simulink model "heli_q8"  (R2024b)
settings: Solver=ode1  StartTime=0.0  StopTime=5  FixedStep=0.002  RelTol=1e-3  EnableMultiTasking=on
PostLoadFcn:
  | qc_set_target_type(getConfigSet(bdroot, 'QUARC Default Target Configuration'));
values from neighbouring files (symbols this model uses):
  A_e = [0 1 0 0 0; 0 0 0 0 0; 0 0 0 1 0; 0 0 0 0 0; K_3 0 0 0 0]    [init_heli_3_10.m]
  Ad = sys_d.A    [init_heli_3_10.m]    (also in midlertidig.m)
  B_e = [0 0; 0 K_1; 0 0; K_2 0; 0 0]    [init_heli_3_10.m]
  Bd = sys_d.B    [init_heli_3_10.m]    (also in midlertidig.m)
  C_e = diag([1 1 1 1 1])    [init_heli_3_10.m]
  Cd = sys_d.C    [init_heli_3_10.m]    (also in midlertidig.m)
  Joystick_gain_x = 1    [init_heli_3_10.m]
  Joystick_gain_y = -1    [init_heli_3_10.m]
  L = place(A_e', C_e', p)'    [init_heli_3_10.m]
  Qd = diag([10^-5, 10^-3, 10^-5, 10^-3, 10^-5, 10^-3])    [init_heli_3_10.m]
  Rh = cov(Yh, 1)    [init_heli_3_10.m]    (also in midlertidig.m)
undefined symbols (not defined in the file or in its folder): HIL, qc_get_step_size
libraries: quarc_library x9
settings Model: SimulationMode=external  ExtModeTrigDuration=5000  Creator=Rchan  LastModifiedBy=Romeo
settings SolverCC: AlgebraicLoopSolver=TrustRegion  PositivePriorityOrder=on
settings DataIOCC: LimitDataPoints=on  SaveFormat=Array  SignalLoggingSaveFormat=ModelDataLogs  ReturnWorkspaceOutputs=off
settings OptimizationCC: ExpressionDepthLimit=2147483647  InitFltsAndDblsToZero=on  LifeSpan=inf
settings DebuggingCC: SaveWithParameterizedLinksMsg=none  UnderspecifiedInitializationDetection=Classic  MergeDetectMultiDrivingBlocksExec=none  SolverPrmCheckMsg=warning  MultiTaskDSMMsg=warning  MultiTaskCondExecSysMsg=none  FcnCallInpInsideContextMsg=warning  UnconnectedInputMsg=warning  UnconnectedOutputMsg=warning  UnconnectedLineMsg=warning  AllowSymbolicDim=off  StateNameClashWarn=warning  SFUnexpectedBacktrackingDiag=warning  SFNoUnconditionalDefaultTransitionDiag=warning  SFExecutionAtInitializationDiag=none  ArithmeticOperatorsInVariantConditions=warning
settings HardwareCC: ProdBitPerPointer=32  ProdBitPerSizeT=32  ProdBitPerPtrDiffT=32  ProdLargestAtomicFloat=None  ProdIntDivRoundTo=Undefined  ProdEndianess=Unspecified  ProdWordSize=32  ProdHWDeviceType=32-bit Generic
settings ModelReferenceCC: EnableRefExpFcnMdlSchedulingChecks=on  PropagateSignalLabelsOutOfModel=off
settings SFSimCC: SimUseLocalCustomCode=off  CustomCodeUndefinedFunction=UseInterfaceOnly
settings RTWCC: Description=QUARC Win64 Target  SystemTargetFile=quarc_win64.tlc  TemplateMakefile=quarc_default_tmf  RTWUseLocalCustomCode=off  GPUComputeCapability=3.5  DLArmComputeVersion=19.05
settings CodeAppCC: StateflowObjectComments=on
settings STFCustomTargetCC: TargetPreCompLibLocation=C:\PROGRA~3\QUARC\lib\2020b\win64\release  ConcurrentExecutionCompliant=on  CPPClassGenCompliant=on  GRTInterface=on  SystemTargetFile=quarc_win64.tlc
settings GRTTargetCC: TargetPreCompLibLocation=C:\PROGRA~3\QUARC\lib\2020b\win64\release  TargetLangStandard=C89/C90 (ANSI)  ParMdlRefBuildCompliant=off  CompOptLevelCompliant=off  CombineOutputUpdateFcns=off  MatFileLogging=off  GRTInterface=on  UseToolchainInfoCompliant=off  ExtMode=on  ExtModeMexFile=quarc_comm
settings ConfigComp: CovMetricSettings=dw  CovSaveCumulativeToWorkspaceVar=on  CovSaveSingleToWorkspaceVar=on  CovExternalEMLEnable=off  CovSFcnEnable=off

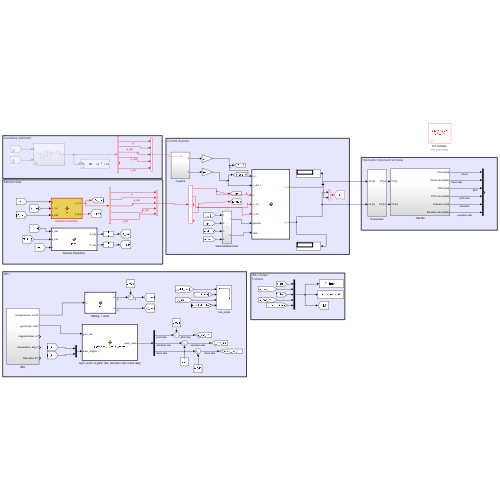
[thumbnail: Simulink's stored preview of the top-level diagram]
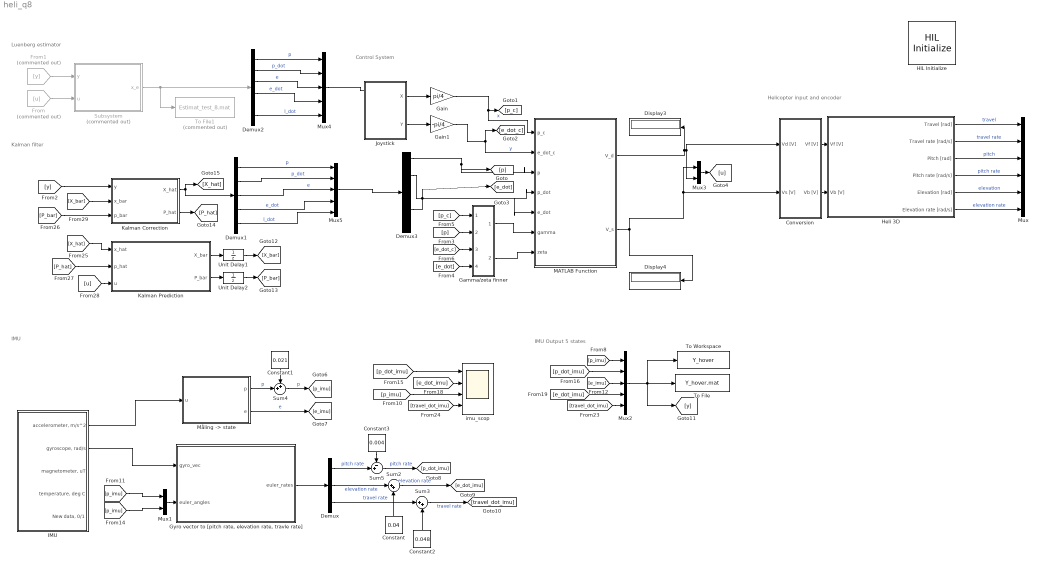
== system heli_q8 ==
  note: Helicopter input and encoder
  note: IMU
  note: Control System
  note: IMU Output
      | 5 states
  note: Kalman filter
  note: Luenberg estimator
  Constant : Constant  Value=0.04
  Constant1 : Constant  Value=0.021
  Constant2 : Constant  Value=0.048
  Constant3 : Constant  Value=0.004
  Conversion : Subsystem
  Demux : Demux  Outputs=3
  Demux1 : Demux  Outputs=5
  Demux2 : Demux  Outputs=6
  Demux3 : Demux  Outputs=5
  Display3 : Display
  Display4 : Display
  From : From  Commented=on  GotoTag=u
  From1 : From  Commented=on  GotoTag=y
  Gain : Gain  Gain=pi/4
  Gain1 : Gain  Gain=-pi/4
  Gamma/zeta finner : Subsystem
  "Gyro vector to [pitch rate, elevation rate, travle rate]" : MATLAB Function  TreatAsAtomicUnit=on
  HIL Initialize : quarc_library/Data Acquisition/Generic/Configuration/HIL Initialize  Priority=-99  object_name=HIL-1  board_type=q8_usb  board_number=0  board_options=update_rate=normal;decimation=1  exclusive=off  active=off  hardware_clocks=[0:2]  clock_modes=[]  initial_clock_frequencies=[]  set_clock_params_at_start=off  set_clock_params_at_switch_in=off  set_clock_frequencies_at_start=off  set_clock_frequencies_at_switch_in=off  analog_input_channels=[0:7]  analog_input_configurations=[]  analog_input_maximums=10  analog_input_minimums=-10  set_analog_input_params_at_start=on  set_analog_input_params_at_switch_in=off  analog_output_channels=[0:7]  analog_output_maximums=10  analog_output_minimums=-10  initial_analog_outputs=[0]  final_analog_outputs=[0]  watchdog_analog_outputs=0  set_analog_output_params_at_start=on  set_analog_output_params_at_switch_in=off  set_analog_outputs_at_start=on  set_analog_outputs_at_switch_in=off  set_analog_outputs_at_terminate=on  set_analog_outputs_at_switch_out=off  set_analog_outputs_on_watchdog=off  digital_input_channels=[]  digital_output_channels=[]  digital_output_configuration=[]  initial_digital_outputs=[1]  final_digital_outputs=[1]  watchdog_digital_outputs=[1]  set_digital_output_params_at_start=off  set_digital_output_params_at_switch_in=off  set_digital_outputs_at_start=on  set_digital_outputs_at_switch_in=off  set_digital_outputs_at_terminate=on  set_digital_outputs_at_switch_out=off  set_digital_outputs_on_watchdog=off  encoder_channels=[0:7]  quadrature=[4]  encoder_filter_frequency=[]  initial_encoder_counts=[0]  set_encoder_params_at_start=on  set_encoder_params_at_switch_in=off  set_encoder_counts_at_start=on  set_encoder_counts_at_switch_in=off  pwm_channels=[0:7]  pwm_modes=0  pwm_frequency=99.532799999999995e6/4095  pwm_configuration=[0]  pwm_alignment=[0]  pwm_polarity=[1]  pwm_leading_deadband=[0]  pwm_trailing_deadband=[0]  initial_pwm_outputs=[0]  final_pwm_outputs=[0]  watchdog_pwm_outputs=[0]  set_pwm_params_at_start=on  set_pwm_params_at_switch_in=off  set_pwm_outputs_at_start=on  set_pwm_outputs_at_switch_in=off  set_pwm_outputs_at_terminate=on  set_pwm_outputs_at_switch_out=off  set_pwm_outputs_on_watchdog=off  other_output_channels=[]  initial_other_outputs=[]  final_other_outputs=[]  watchdog_other_outputs=[]  set_other_outputs_at_start=off  set_other_outputs_at_switch_in=off  set_other_outputs_at_terminate=off  set_other_outputs_at_switch_out=off  set_other_outputs_on_watchdog=off
  Heli 3D : Subsystem
  IMU : Subsystem
  Joystick : Subsystem
  Kalman Correction : MATLAB Function  TreatAsAtomicUnit=on
  Kalman Prediction : MATLAB Function  TreatAsAtomicUnit=on
  MATLAB Function : MATLAB Function  TreatAsAtomicUnit=on
  Mux : Mux  Inputs=6
  Mux1 : Mux  Inputs=2
  Mux2 : Mux  Inputs=5
  Mux3 : Mux  Inputs=2
  Mux4 : Mux  Inputs=5
  Mux5 : Mux  Inputs=5
  "Måling -> state" : MATLAB Function  TreatAsAtomicUnit=on
  Subsystem : Subsystem  Commented=on
  Sum2 : Sum  Inputs=|++
  Sum3 : Sum  Inputs=|++
  Sum4 : Sum  Inputs=++|
  Sum5 : Sum  Inputs=-+|
  To File : ToFile  Filename=Y_hover.mat
  To File1 : ToFile  Commented=on  Filename=Estimat_test_8.mat
  To Workspace : ToWorkspace  VariableName=Y_hover  SampleTime=-1
  Unit Delay1 : UnitDelay  InitialCondition=[0; 0; 0; 0; 0; 0]  SampleTime=-1  HasFrameUpgradeWarning=on
  Unit Delay2 : UnitDelay  InitialCondition=[0 0 0 0 0 0; 0 0 0 0 0 0; 0 0 0 0 0 0; 0 0 0 0 0 0; 0 0 0 0 0 0; 0 0 0 0 0 0]  SampleTime=-1  HasFrameUpgradeWarning=on
  imu_scop : Scope  NumInputPorts=4
  wires:
  Heli 3D/1(Travel [rad]) -> Mux/1  "travel"
  Heli 3D/3(Pitch [rad]) -> Mux/3  "pitch"
  Heli 3D/4(Pitch rate [rad/s]) -> Mux/4  "pitch rate"
  Heli 3D/6(Elevation rate [rad/s]) -> Mux/6  "elevation rate"
  Joystick/1(X) -> Gain/1
  Joystick/2(Y) -> Gain1/1
  Gain1/1 -> [e_dot_c], MATLAB Function/2(e_dot_c)  "y"
  Gain/1 -> MATLAB Function/1(p_c), [p_c]  "x"
  Heli 3D/5(Elevation [rad]) -> Mux/5  "elevation"
  MATLAB Function/1(V_d) -> Conversion/1(Vd [V]), Mux3/2, Display3/1
  MATLAB Function/2(V_s) -> Mux3/1, Conversion/2(Vs [V]), Display4/1
  IMU/1("accelerometer, m/s^2") -> "Måling -> state"/1(u)
  IMU/2("gyroscope, rad/s") -> "Gyro vector to [pitch rate, elevation rate, travle rate]"/1(gyro_vec)
  "Måling -> state"/2(e) -> [e_imu]  "e"
  Mux1/1 -> "Gyro vector to [pitch rate, elevation rate, travle rate]"/2(euler_angles)
  "Gyro vector to [pitch rate, elevation rate, travle rate]"/1(euler_rates) -> Demux/1
  Heli 3D/2(Travel rate [rad/s]) -> Mux/2  "travel rate"
  Conversion/1(Vf [V]) -> Heli 3D/1(Vf [V])
  Conversion/2(Vb [V]) -> Heli 3D/2(Vb [V])
  Subsystem/1(x_e) -> Demux2/1, To File1/1
  Demux3/1 -> MATLAB Function/3(p), [p]
  Demux3/2 -> MATLAB Function/4(p_dot)
  Demux3/4 -> [e_dot], MATLAB Function/5(e_dot)
  Mux3/1 -> [u]
  From/1 -> Subsystem/2(u)
  From1/1 -> Subsystem/1(y)
  Sum4/1 -> [p_imu]  "p"
  Mux2/1 -> To Workspace/1, To File/1, [y]
  Demux/2 -> Sum2/1  "elevation rate"
  Sum2/1 -> [e_dot_imu]  "elevation rate"
  Constant/1 -> Sum2/2
  Demux/3 -> Sum3/1  "travel rate"
  Sum3/1 -> [travel_dot_imu]  "travel rate"
  Constant2/1 -> Sum3/2
  Demux/1 -> Sum5/2  "pitch rate"
  Sum5/1 -> [p_dot_imu]  "pitch rate"
  "Måling -> state"/1(p) -> Sum4/2  "p"
  Constant1/1 -> Sum4/1
  Constant3/1 -> Sum5/1
  Demux1/1 -> Mux5/1  "p"
  Demux1/2 -> Mux5/2  "p_dot"
  Demux1/3 -> Mux5/3  "e"
  Demux1/4 -> Mux5/4  "e_dot"
  Demux1/5 -> Mux5/5  "l_dot"
  [y] -> Kalman Correction/1(y)
  Gamma/zeta finner/1(Out1) -> MATLAB Function/6(gamma)
  Gamma/zeta finner/2(Out2) -> MATLAB Function/7(zeta)
  [p] -> Gamma/zeta finner/2(In2)
  [e_dot] -> Gamma/zeta finner/4(In4)
  [p_c] -> Gamma/zeta finner/1(In1)
  [e_dot_c] -> Gamma/zeta finner/3(In3)
  [p_imu] -> Mux2/1
  [p_imu] -> imu_scop/3
  [p_imu] -> Mux1/1
  [e_imu] -> Mux2/3
  [p_imu] -> Mux1/2
  [p_dot_imu] -> imu_scop/1
  [p_dot_imu] -> Mux2/2
  [e_dot_imu] -> imu_scop/2
  [e_dot_imu] -> Mux2/4
  [travel_dot_imu] -> Mux2/5
  [travel_dot_imu] -> imu_scop/4
  Kalman Correction/1(X_hat) -> [X_hat], Demux1/1
  Kalman Correction/2(P_hat) -> [P_hat]
  [X_bar] -> Kalman Correction/2(x_bar)
  [P_bar] -> Kalman Correction/3(p_bar)
  Kalman Prediction/1(X_bar) -> Unit Delay1/1
  Kalman Prediction/2(P_bar) -> Unit Delay2/1
  Unit Delay2/1 -> [P_bar]
  [X_hat] -> Kalman Prediction/1(x_hat)
  [P_hat] -> Kalman Prediction/2(p_hat)
  [u] -> Kalman Prediction/3(u)
  Mux5/1 -> Demux3/1
  Unit Delay1/1 -> [X_bar]
  Demux2/4 -> Mux4/4  "e_dot"
  Demux2/1 -> Mux4/1  "p"
  Demux2/2 -> Mux4/2  "p_dot"
  Mux4/1 -> ?
  Demux2/6 -> Mux4/5  "l_dot"
  Demux2/3 -> Mux4/3  "e"

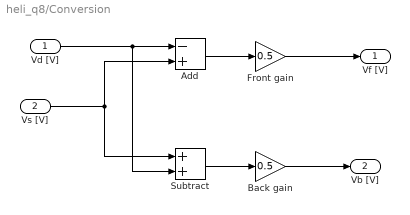
== system heli_q8/Conversion ==
  Vd [V] : Inport
  Vs [V] : Inport  Port=2
  Add : Sum  Inputs=-+
  Back gain : Gain  Gain=0.5
  Front gain : Gain  Gain=0.5
  Subtract : Sum
  Vf [V] : Outport
  Vb [V] : Outport  Port=2
  wires:
  Vd [V]/1 -> Subtract/2, Add/1
  Vs [V]/1 -> Subtract/1, Add/2
  Subtract/1 -> Back gain/1
  Back gain/1 -> Vb [V]/1
  Add/1 -> Front gain/1
  Front gain/1 -> Vf [V]/1

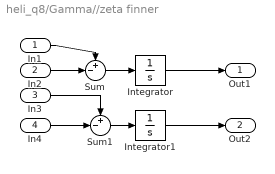
== system heli_q8/Gamma//zeta finner ==
  In1 : Inport
  In2 : Inport  Port=2
  In3 : Inport  Port=3
  In4 : Inport  Port=4
  Integrator : Integrator
  Integrator1 : Integrator
  Sum : Sum  Inputs=+-|
  Sum1 : Sum  Inputs=+-|
  Out1 : Outport
  Out2 : Outport  Port=2
  wires:
  Sum1/1 -> Integrator1/1
  Sum/1 -> Integrator/1
  In3/1 -> Sum1/1
  In1/1 -> Sum/1
  Integrator/1 -> Out1/1
  Integrator1/1 -> Out2/1
  In2/1 -> Sum/2
  In4/1 -> Sum1/2

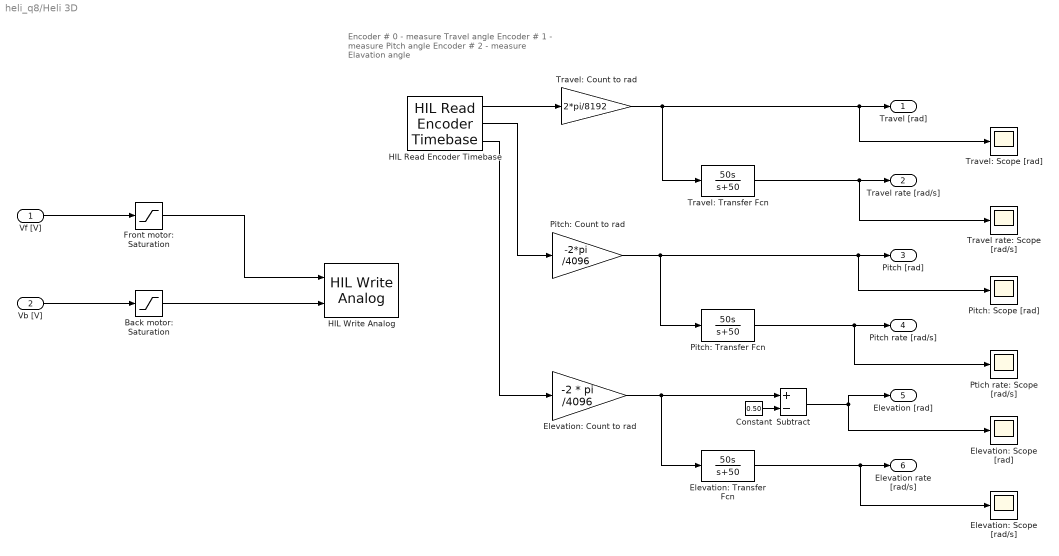
== system heli_q8/Heli 3D ==
  note: Encoder # 0 - measure Travel angle
      | Encoder # 1 - measure Pitch angle
      | Encoder # 2 - measure Elavation angle
  Vf [V] : Inport
  Vb [V] : Inport  Port=2
  Back motor: Saturation : Saturate  UpperLimit=5  LowerLimit=-5
  Constant : Constant  Value=0.50
  Elevation: Count to rad : Gain  Gain=-2 * pi /4096
  Elevation: Scope [rad/s] : Scope
  Elevation: Scope [rad] : Scope
  Elevation: Transfer Fcn : TransferFcn  Numerator=[50 0]  Denominator=[1 50]
  Front motor: Saturation : Saturate  UpperLimit=5  LowerLimit=-5
  HIL Read Encoder Timebase : quarc_library/Data Acquisition/Generic/Timebases/HIL Read Encoder Timebase  object_name=HIL-1  clock=0  channels=[0:2]  active=on  vector_output=off  data_type_mode=Inherit via back propagation  data_type=double  overflow_mode=Error on overflow  samples_in_buffer=max(ceil(1/qc_get_step_size), 1)
  HIL Write Analog : quarc_library/Data Acquisition/Generic/Immediate I//O/HIL Write Analog  object_name=HIL-1  channels=[0:1]  sample_time=-1  active=off  vector_input=off
  Pitch: Count to rad : Gain  Gain=-2*pi /4096
  Pitch: Scope [rad] : Scope
  Pitch: Transfer Fcn : TransferFcn  Numerator=[50 0]  Denominator=[1 50]
  Ptich rate: Scope [rad/s] : Scope
  Subtract : Sum  Inputs=+-
  Travel rate: Scope [rad/s] : Scope
  Travel: Count to rad : Gain  Gain=2*pi/8192
  Travel: Scope [rad] : Scope
  Travel: Transfer Fcn : TransferFcn  Numerator=[50 0]  Denominator=[1 50]
  Travel [rad] : Outport
  Travel rate [rad/s] : Outport  Port=2
  Pitch [rad] : Outport  Port=3
  Pitch rate [rad/s] : Outport  Port=4
  Elevation [rad] : Outport  Port=5
  Elevation rate [rad/s] : Outport  Port=6
  wires:
  HIL Read Encoder Timebase/1 -> Travel: Count to rad/1
  HIL Read Encoder Timebase/2 -> Pitch: Count to rad/1
  HIL Read Encoder Timebase/3 -> Elevation: Count to rad/1
  Travel: Count to rad/1 -> Travel: Scope [rad]/1, Travel [rad]/1, Travel: Transfer Fcn/1
  Travel: Transfer Fcn/1 -> Travel rate: Scope [rad/s]/1, Travel rate [rad/s]/1
  Pitch: Count to rad/1 -> Pitch: Transfer Fcn/1, Pitch: Scope [rad]/1, Pitch [rad]/1
  Pitch: Transfer Fcn/1 -> Ptich rate: Scope [rad/s]/1, Pitch rate [rad/s]/1
  Elevation: Transfer Fcn/1 -> Elevation: Scope [rad/s]/1, Elevation rate [rad/s]/1
  Vf [V]/1 -> Front motor: Saturation/1
  Vb [V]/1 -> Back motor: Saturation/1
  Front motor: Saturation/1 -> HIL Write Analog/1
  Back motor: Saturation/1 -> HIL Write Analog/2
  Constant/1 -> Subtract/2
  Elevation: Count to rad/1 -> Subtract/1, Elevation: Transfer Fcn/1
  Subtract/1 -> Elevation: Scope [rad]/1, Elevation [rad]/1

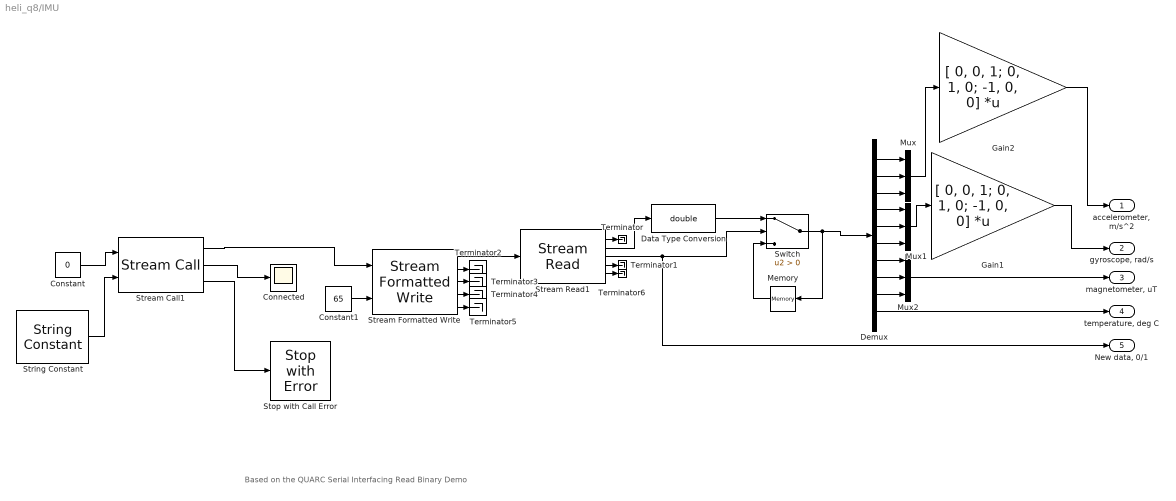
== system heli_q8/IMU ==
  note: Based on the QUARC Serial Interfacing Read Binary Demo
  Connected : Scope
  Constant : Constant  Value=0
  Constant1 : Constant  Value=65
  Data Type Conversion : DataTypeConversion  OutDataTypeStr=double  SaturateOnIntegerOverflow=off  RndMeth=Floor
  Demux : Demux  Outputs=10
  Gain1 : Gain  Gain=[ 0, 0, 1; 0, 1, 0; -1, 0, 0]  Multiplication=Matrix(K*u) (u vector)
  Gain2 : Gain  Gain=[ 0, 0, 1; 0, 1, 0; -1, 0, 0]  Multiplication=Matrix(K*u) (u vector)
  Memory : Memory  InitialCondition=[0 0 0 0 0 0 0 0 0 0]
  Mux : Mux  Inputs=3
  Mux1 : Mux  Inputs=3
  Mux2 : Mux  Inputs=3
  Stop with Call Error : quarc_library/Sinks/Error Handling/Stop with Error  message_type=Interpret input as error code  message=Error occurred
      settings: SourceProductName=QUARC Targets
  Stream Call1 : quarc_library/Communications/Intermediate/Stream Call  uri_source=External input port  uri=serial://IMU:9?baud=115200,word=8,parity=none,stop=1,flow='none'  apply_uri_to_all_configs=on  send_buffer_size=8000  receive_buffer_size=8000  byte_order=little endian (Intel - LSB first)  sample_time=qc_get_step_size  non_blocking=on  active=off
      settings: SourceProductName=QUARC Targets
  Stream Formatted Write : quarc_library/Communications/Intermediate/Stream Formatted Write  format_string=%c\n  max_code_units=80  optimization=Minimizing latency
      settings: SourceProductName=QUARC Targets
  Stream Read1 : quarc_library/Communications/Intermediate/Stream Read  data_type=single  type_expr=BusObject  num_elements=10  receive_dims=off
      settings: SourceProductName=QUARC Targets
  String Constant : quarc_library/Strings/String Constant  string_value=qc_perform_substitutions('serial://IMU:%{PORT}?baud=115200,word=8,parity=none,stop=1')  evaluate_string=on  string_type=URI  max_length=255  sample_time=inf  variable_size=off
      settings: AttributesFormatString="\"serial://IMU:3?baud=115200,word=8,parity=none,stop=1\""  SourceProductName=QUARC Targets
  Switch : Switch  Criteria=u2 > Threshold  SaturateOnIntegerOverflow=off  InputSameDT=off
  Terminator{,1..6} (7 alike) : Terminator
  "accelerometer, m/s^2" : Outport
  "gyroscope, rad/s" : Outport  Port=2
  "magnetometer, uT" : Outport  Port=3
  "temperature, deg C" : Outport  Port=4
  "New data, 0/1" : Outport  Port=5
  wires:
  Switch/1 -> Memory/1, Demux/1
  Data Type Conversion/1 -> Switch/1
  Stream Read1/3 -> "New data, 0/1"/1, Switch/2
  Stream Formatted Write/1 -> Stream Read1/1
  Constant1/1 -> Stream Formatted Write/2
  Gain1/1 -> "gyroscope, rad/s"/1
  Gain2/1 -> "accelerometer, m/s^2"/1
  Stream Read1/4 -> Terminator1/1
  Demux/10 -> "temperature, deg C"/1
  Mux1/1 -> Gain1/1
  Stream Read1/2 -> Data Type Conversion/1
  Demux/7 -> Mux2/1
  Demux/8 -> Mux2/2
  Demux/9 -> Mux2/3
  Mux2/1 -> "magnetometer, uT"/1
  Demux/6 -> Mux1/3
  Demux/5 -> Mux1/2
  Demux/4 -> Mux1/1
  Mux/1 -> Gain2/1
  Demux/3 -> Mux/3
  Demux/1 -> Mux/1
  Demux/2 -> Mux/2
  Stream Read1/1 -> Terminator/1
  Stream Call1/1 -> Stream Formatted Write/1
  Constant/1 -> Stream Call1/1
  String Constant/1 -> Stream Call1/2
  Stream Call1/2 -> Connected/1
  Stream Call1/3 -> Stop with Call Error/1
  Memory/1 -> Switch/3
  Stream Formatted Write/2 -> Terminator2/1
  Stream Formatted Write/3 -> Terminator3/1
  Stream Formatted Write/4 -> Terminator4/1
  Stream Formatted Write/5 -> Terminator5/1
  Stream Read1/5 -> Terminator6/1

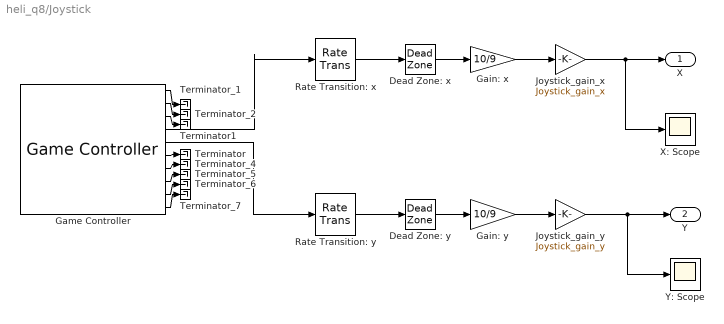
== system heli_q8/Joystick ==
  Dead Zone: x : DeadZone  LowerValue=-0.1  UpperValue=0.1
  Dead Zone: y : DeadZone  LowerValue=-0.1  UpperValue=0.1
  Gain: x : Gain  Gain=10/9
  Gain: y : Gain  Gain=10/9
  Game Controller : quarc_library/Devices/Peripherals/Target/Game Controller  controller=1  buffer_size=12  deadzone=[]  saturation=[]  sample_time=max(qc_get_step_size, 0.01)  auto_center=off  enabled=on
      settings: SourceProductName=QUARC Targets
  Joystick_gain_x : Gain  Gain=Joystick_gain_x
  Joystick_gain_y : Gain  Gain=Joystick_gain_y
  Rate Transition: x : RateTransition
  Rate Transition: y : RateTransition
  Terminator : Terminator
  Terminator1 : Terminator
  Terminator_{1..2,4..7} (6 alike) : Terminator
  X: Scope : Scope
  Y: Scope : Scope
  X : Outport
  Y : Outport  Port=2
  wires:
  Rate Transition: y/1 -> Dead Zone: y/1
  Rate Transition: x/1 -> Dead Zone: x/1
  Game Controller/5 -> Rate Transition: y/1
  Game Controller/4 -> Rate Transition: x/1
  Game Controller/1 -> Terminator_1/1
  Game Controller/2 -> Terminator_2/1
  Game Controller/7 -> Terminator_4/1
  Game Controller/8 -> Terminator_5/1
  Game Controller/9 -> Terminator_6/1
  Game Controller/10 -> Terminator_7/1
  Game Controller/3 -> Terminator1/1
  Game Controller/6 -> Terminator/1
  Dead Zone: x/1 -> Gain: x/1
  Dead Zone: y/1 -> Gain: y/1
  Gain: x/1 -> Joystick_gain_x/1
  Gain: y/1 -> Joystick_gain_y/1
  Joystick_gain_x/1 -> X/1, X: Scope/1
  Joystick_gain_y/1 -> Y: Scope/1, Y/1

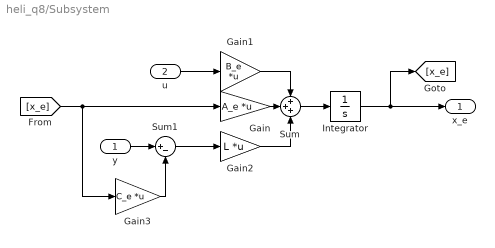
== system heli_q8/Subsystem ==
  y : Inport
  u : Inport  Port=2
  Gain : Gain  Gain=A_e  Multiplication=Matrix(K*u)
  Gain1 : Gain  Gain=B_e  Multiplication=Matrix(K*u)
  Gain2 : Gain  Gain=L  Multiplication=Matrix(K*u)
  Gain3 : Gain  Gain=C_e  Multiplication=Matrix(K*u)
  Integrator : Integrator
  Sum : Sum  Inputs=+++
  Sum1 : Sum  Inputs=|+-
  x_e : Outport
  wires:
  Gain/1 -> Sum/2
  u/1 -> Gain1/1
  Gain1/1 -> Sum/1
  Gain2/1 -> Sum/3
  Sum/1 -> Integrator/1
  Integrator/1 -> [x_e], x_e/1
  [x_e] -> Gain3/1, Gain/1
  Sum1/1 -> Gain2/1
  y/1 -> Sum1/1
  Gain3/1 -> Sum1/2

== matlab function heli_q8/Gyro vector to [pitch rate, elevation rate, travle rate] ==
  data: gyro_vec input; euler_rates output; euler_angles input
function euler_rates = gyro_vec_to_euler_rates(gyro_vec,euler_angles)
%#codegen
    phi = euler_angles(1);
    theta = euler_angles(2);
    %psi = euler_angles(3);


    T = [1, sin(phi)*tan(theta), cos(phi)*tan(theta);
         0, cos(phi),            -sin(phi);
         0, sin(phi)/cos(theta), cos(phi)/cos(theta)]; 
euler_rates = T*gyro_vec;

== matlab function heli_q8/MATLAB Function ==
  data: V_d output; p_c input; V_s output; e_dot_c input; p input; p_dot input; e_dot input; gamma input; zeta input; K parameter
function [V_d, V_s] = fcn(p_c, e_dot_c, p, p_dot, e_dot, gamma, zeta, K)

F = [K(1, 1) K(1, 3); K(2, 1) K(2, 3)];

u = F*[p_c; e_dot_c]-K*[p; p_dot; e_dot; gamma; zeta];

V_s = u(1, 1) + 7.5;
V_d = u(2, 1);

== matlab function heli_q8/Måling -> state ==
  data: u input; p output; e output
function [p,e] = fcn(u)

ax = u(1);
ay = u(2);
az = u(3);

if ax == 0
    ax = eps;
end

if ay == 0
    ay = eps;
end

if az == 0
    az = eps;
end

p = atan(ay/az);
e = atan(ax/(sqrt(ay^2+az^2)));

== matlab function heli_q8/Kalman Correction ==
  data: X_hat output; y input; Cd parameter; Rh parameter; x_bar input; P_hat output; p_bar input
function [X_hat, P_hat] = cor(y, Cd, Rh, x_bar, p_bar)

% if isempty(x_bar)
%     I = diag([1 1 1 1 1 1]);
%     x_bar = [0; 0; 0; 0; 0; 0];
%     p_bar = [0 0 0 0 0 0; 0 0 0 0 0 0; 0 0 0 0 0 0; 0 0 0 0 0 0; 0 0 0 0 0 0; 0 0 0 0 0 0];
% end

L = p_bar * transpose(Cd) * (Cd * p_bar * transpose(Cd) + Rh)^(-1); 
x_hat = x_bar + L * (y - Cd * x_bar);
p_hat = (I - L * Cd) * p_bar * transpose(I - L * Cd) + L * Rh * transpose(L);

X_hat = x_hat;
P_hat = p_hat;
end

== matlab function heli_q8/Kalman Prediction ==
  data: x_hat input; p_hat input; u input; X_bar output; P_bar output; Ad parameter; Qd parameter; Bd parameter
function [X_bar, P_bar] = pred(x_hat, p_hat, u, Ad, Qd, Bd)

X_bar = Ad * x_hat + Bd * u;
P_bar = Ad * p_hat * transpose(Ad) + Qd;

end
